simulink model "rlDronePidTuning"  (R2024b)
settings: Solver=VariableStepAuto  StartTime=0.0  StopTime=60  RelTol=1e-3
libraries: simulink x5, rllib x1
settings Model: Creator=Feder  LastModifiedBy=Alessandro
settings DataIOCC: ReturnWorkspaceOutputs=off
settings DebuggingCC: AlgebraicLoopMsg=none

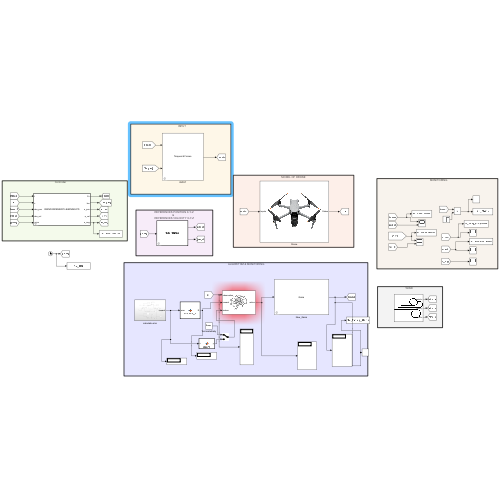
[thumbnail: Simulink's stored preview of the top-level diagram]
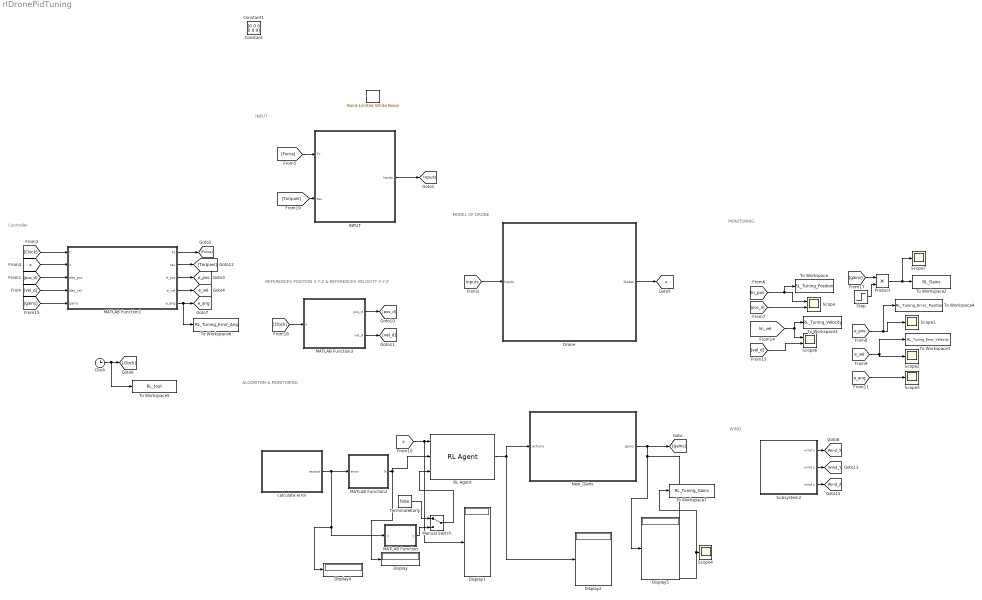
== system rlDronePidTuning ==
  note: MONITORING
  note: ALGORITHM & MONITORING
  note: Controller
  note: REFERENCES POSITION X-Y-Z
      |                                                 &
      |                         REFERENCES VELOCITY X-Y-Z
  note: INPUT
  note: MODEL OF DRONE
  note: WIND
  Clock : Clock
  Display{,1..2,4..5} (5 alike) : Display
  Drone : Subsystem
      mask Display: image('DJI Air 3S.png');
  INPUT : Subsystem
      mask Display: disp('Torques & Forces');
  MATLAB Function : MATLAB Function  TreatAsAtomicUnit=on
  MATLAB Function1 : MATLAB Function  TreatAsAtomicUnit=on
  MATLAB Function2 : MATLAB Function  TreatAsAtomicUnit=on
  MATLAB Function3 : MATLAB Function  TreatAsAtomicUnit=on
  Manual Switch : ManualSwitch
  New_Gains : Subsystem
      mask Display: disp('Gains');
  Product : Product
  RL Agent : rllib/RL Agent  Agent=myAgent  ExternalActionAsInput=off  ProvideLastAction=off  ProvideCumRwd=off  TreatAsDirectFeedthrough=on  UseStrictObservationDataTypes=off
  Scope : Scope  NumInputPorts=2
  Scope{1..4,7} (5 alike) : Scope
  Scope6 : Scope  NumInputPorts=2
  Step : Step  Time=0  SampleTime=0
  Subsystem2 : Subsystem
      mask Display: image('wind-14.png');
  TerminateEarly : Constant  Value=false
  To Workspace : ToWorkspace  VariableName=RL_Tuning_Position  SampleTime=-1
  To Workspace1 : ToWorkspace  VariableName=RL_Tuning_Velocity  SampleTime=-1
  To Workspace2 : ToWorkspace  VariableName=RL_Gains  SampleTime=-1
  To Workspace3 : ToWorkspace  VariableName=RL_Tuning_Error_Velocity  SampleTime=-1
  To Workspace4 : ToWorkspace  VariableName=RL_Tuning_Error_Position  SampleTime=-1
  To Workspace5 : ToWorkspace  VariableName=RL_tout  SampleTime=-1
  To Workspace6 : ToWorkspace  VariableName=RL_Tuning_Error_Ang  SampleTime=-1
  To Workspace7 : ToWorkspace  VariableName=RL_Tuning_Gains  SaveFormat=Timeseries  SampleTime=-1
  calculate error : Subsystem
  " " : simulink/Sources/Band-Limited White Noise  IOType=siggen  Cov=[0.1]  Ts=0.1  seed=[23341]
      settings: LibrarySourceBlock=|
      | simgens/Band-Limited
      | White Noise
  Constant : Constant  IOType=siggen
  Constant1 : Constant  IOType=siggen  Value=[0 0 0 0 0 0]
  tag scope: Inputs=global, Wind_X=global, Wind_Y=global, Wind_Z=global, e_ang=global, e_pos=global, e_vel=global, x=global
  wires:
  MATLAB Function1/3(e_pos) -> [e_pos]
  MATLAB Function1/4(e_vel) -> [e_vel]
  [x] -> MATLAB Function1/2(x)
  [vel_d] -> MATLAB Function1/4(des_vel)
  [pos_d] -> MATLAB Function1/3(des_pos)
  Clock/1 -> To Workspace5/1, [Clock]
  [Clock] -> MATLAB Function1/1(t)
  [lin_pos] -> Scope/1, To Workspace/1
  [pos_d] -> Scope/2
  MATLAB Function2/1(R) -> Display/1, RL Agent/2
  [x] -> Display1/1, RL Agent/1
  [vel_d] -> Scope6/2
  [lin_vel] -> To Workspace1/1, Scope6/1
  Step/1 -> Product/2
  Product/1 -> To Workspace2/1, Scope7/1
  [gains] -> MATLAB Function1/5(gains)
  [gains] -> Product/1
  [e_pos] -> To Workspace4/1, Scope1/1
  [e_vel] -> To Workspace3/1, Scope2/1
  [e_ang] -> Scope3/1
  [Clock] -> MATLAB Function3/1(t)
  MATLAB Function3/2(vel_d) -> [vel_d]
  MATLAB Function3/1(pos_d) -> [pos_d]
  [Force] -> INPUT/1(Fz)
  [Torques] -> INPUT/2(tau)
  INPUT/1(Inputs) -> [Inputs]
  MATLAB Function1/1(Fz) -> [Force]
  MATLAB Function1/2(tau) -> [Torques]
  MATLAB Function1/5(e_ang) -> To Workspace6/1, [e_ang]
  Drone/1(States) -> [x]
  [Inputs] -> Drone/1(Inputs)
  Subsystem2/2(wind y) -> [Wind_Y]
  Subsystem2/1(wind x) -> [Wind_X]
  Subsystem2/3(wind z) -> [Wind_Z]
  New_Gains/1(gains) -> [gains], To Workspace7/1, Scope4/1, Display5/1
  RL Agent/1 -> Display2/1, New_Gains/1(actions)
  calculate error/1(reward) -> MATLAB Function/1(u), Display4/1, MATLAB Function2/1(error)
  TerminateEarly/1 -> Manual Switch/1
  MATLAB Function/1(y) -> Manual Switch/2
  Manual Switch/1 -> RL Agent/3

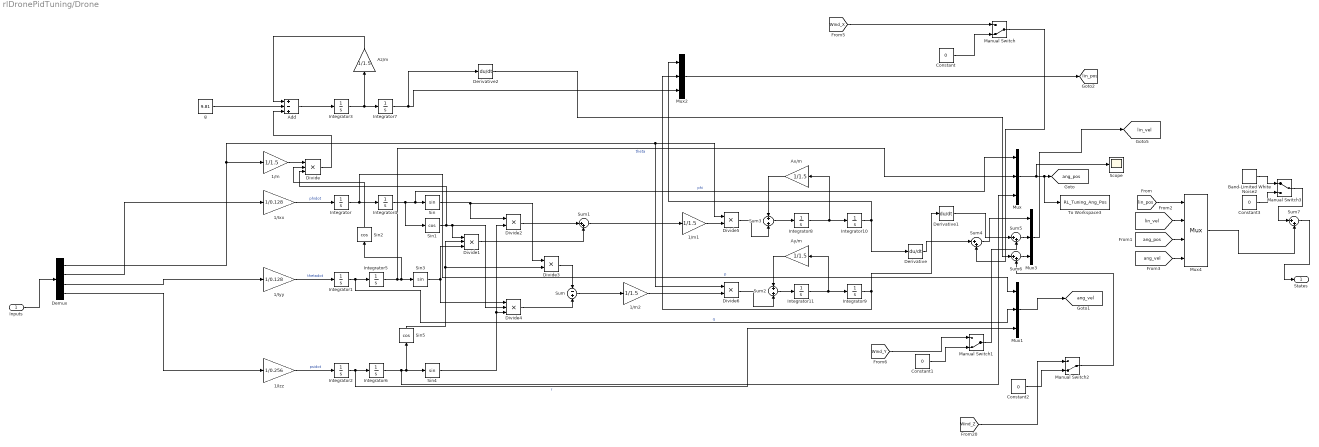
== system rlDronePidTuning/Drone ==
  Inputs : Inport
  1/Ixx : Gain  Gain=1/0.128
  1/Iyy : Gain  Gain=1/0.128
  1/Izz : Gain  Gain=1/0.256
  1/m : Gain  Gain=1/1.5
  1/m1 : Gain  Gain=1/1.5
  1/m2 : Gain  Gain=1/1.5
  Add : Sum  Inputs=+-+
  Ax/m : Gain  Gain=1/1.5
  Ay/m : Gain  Gain=1/1.5
  Az/m : Gain  Gain=1/1.5
  Band-Limited White Noise2 : simulink/Sources/Band-Limited White Noise  Cov=[0.00001]  Ts=0.01  seed=[23341]
  Constant{,1..3} (4 alike) : Constant  Value=0
  Demux : Demux
  Derivative : Derivative
  Derivative1 : Derivative
  Derivative2 : Derivative
  Divide : Product  Inputs=***
  Divide1 : Product  Inputs=***
  Divide{2..3,5..6} (4 alike) : Product  Inputs=**
  Divide4 : Product  Inputs=***
  Integrator{,1..11} (12 alike) : Integrator
  Manual Switch : ManualSwitch  CurrentSetting=0
  Manual Switch1 : ManualSwitch  CurrentSetting=0
  Manual Switch2 : ManualSwitch  CurrentSetting=0
  Manual Switch3 : ManualSwitch
  Mux{,1..3} (4 alike) : Mux  Inputs=3
  Mux4 : Mux
  Scope : Scope
  Sin : Trigonometry
  Sin1 : Trigonometry  Operator=cos
  Sin2 : Trigonometry  Operator=cos
  Sin3 : Trigonometry
  Sin4 : Trigonometry
  Sin5 : Trigonometry  Operator=cos
  Sum : Sum  Inputs=-+
  Sum{1,4..7} (5 alike) : Sum  Inputs=|++
  Sum2 : Sum
  Sum3 : Sum
  To Workspace3 : ToWorkspace  VariableName=RL_Tuning_Ang_Pos  SampleTime=-1
  g : Constant  Value=9.81
  States : Outport
  tag scope: ang_pos=global, ang_vel=global, lin_pos=global, lin_vel=global
  wires:
  Ay/m/1 -> Sum2/1
  Sum3/1 -> Integrator8/1
  Divide2/1 -> Sum1/1
  Integrator5/1 -> Mux/2, Sin2/1, Sin3/1  "theta"
  Ax/m/1 -> Sum3/1
  Integrator2/1 -> Mux1/3, Integrator6/1  "r"
  Demux/1 -> Divide6/1, Divide5/1, 1/m/1
  Integrator11/1 -> Ay/m/1, Integrator9/1
  Divide1/1 -> Sum1/2
  1/Izz/1 -> Integrator2/1  "psidot"
  Divide6/1 -> Sum2/2
  Divide5/1 -> Sum3/2
  Sum/1 -> 1/m2/1
  Integrator6/1 -> Mux/3, Sin5/1, Sin4/1
  Az/m/1 -> Add/1
  Integrator3/1 -> Az/m/1, Integrator7/1
  Divide/1 -> Add/3
  Integrator/1 -> Mux1/1, Integrator4/1  "p"
  Sin4/1 -> Divide2/2, Divide4/3
  Integrator10/1 -> Mux2/1, Derivative/1
  Divide4/1 -> Sum/2
  1/Ixx/1 -> Integrator/1  "phidot"
  Add/1 -> Integrator3/1
  Integrator9/1 -> Derivative1/1, Mux2/2
  Divide3/1 -> Sum/1
  1/Iyy/1 -> Integrator1/1  "thetadot"
  Sin/1 -> Divide2/1, Divide3/1
  1/m2/1 -> Divide6/2
  Integrator1/1 -> Mux1/2, Integrator5/1  "q"
  Sin2/1 -> Divide/2
  Sin5/1 -> Divide1/2, Divide3/2
  Sum2/1 -> Integrator11/1
  Integrator4/1 -> Mux/1, Sin/1, Sin1/1  "phi"
  Sin1/1 -> Divide/3, Divide1/1, Divide4/2
  g/1 -> Add/2
  1/m/1 -> Divide/1
  Sin3/1 -> Divide4/1, Divide1/3
  Sum1/1 -> 1/m1/1
  1/m1/1 -> Divide5/2
  Integrator8/1 -> Ax/m/1, Integrator10/1
  Mux/1 -> Scope/1, To Workspace3/1, [ang_pos]
  Mux1/1 -> [ang_vel]
  Integrator7/1 -> Derivative2/1, Mux2/3
  [lin_pos] -> Mux4/1
  [ang_pos] -> Mux4/3
  [lin_vel] -> Mux4/2
  [ang_vel] -> Mux4/4
  Demux/2 -> 1/Ixx/1
  Demux/3 -> 1/Iyy/1
  Demux/4 -> 1/Izz/1
  Inputs/1 -> Demux/1
  Mux2/1 -> [lin_pos]
  Mux3/1 -> [lin_vel]
  [Wind_X] -> Manual Switch/1
  Constant/1 -> Manual Switch/2
  Manual Switch/1 -> Sum4/2
  Derivative/1 -> Sum4/1
  Sum4/1 -> Mux3/1
  Derivative1/1 -> Sum5/1
  Sum5/1 -> Mux3/2
  Constant1/1 -> Manual Switch1/2
  [Wind_Y] -> Manual Switch1/1
  Manual Switch1/1 -> Sum5/2
  Sum6/1 -> Mux3/3
  Derivative2/1 -> Sum6/1
  [Wind_Z] -> Manual Switch2/1
  Constant2/1 -> Manual Switch2/2
  Manual Switch2/1 -> Sum6/2
  Sum7/1 -> States/1
  Mux4/1 -> Sum7/2
  Band-Limited White Noise2/1 -> Manual Switch3/1
  Constant3/1 -> Manual Switch3/2
  Manual Switch3/1 -> Sum7/1

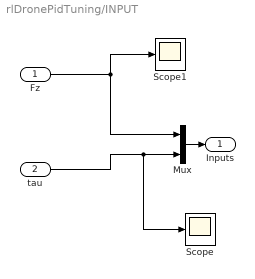
== system rlDronePidTuning/INPUT ==
  Fz : Inport
  tau : Inport  Port=2
  Mux : Mux  Inputs=2
  Scope : Scope
  Scope1 : Scope
  Inputs : Outport
  wires:
  Fz/1 -> Mux/1, Scope1/1
  Mux/1 -> Inputs/1
  tau/1 -> Scope/1, Mux/2

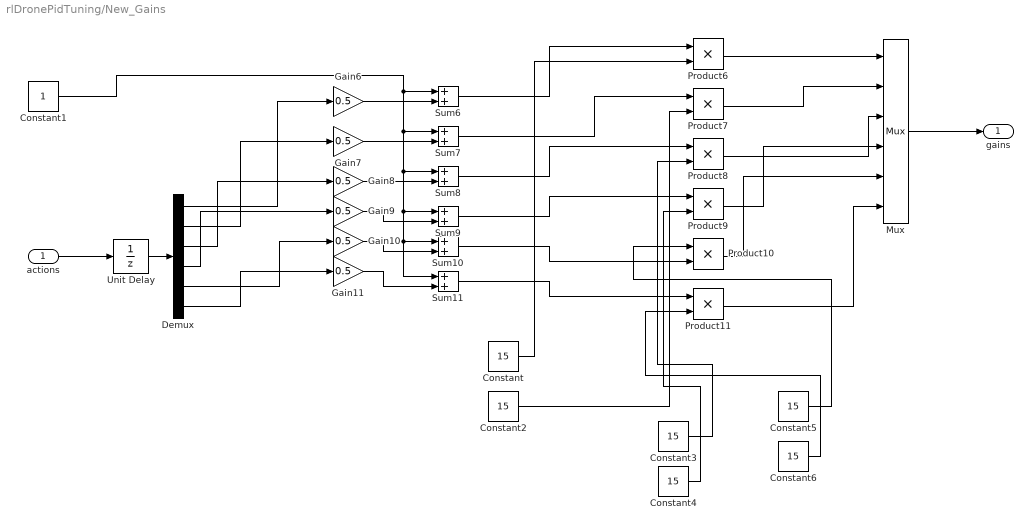
== system rlDronePidTuning/New_Gains ==
  actions : Inport
  Constant{,2..6} (6 alike) : Constant  Value=15
  Constant1 : Constant
  Demux : Demux  Outputs=6
  Gain{6..11} (6 alike) : Gain  Gain=0.5
  Mux : Mux  Inputs=6
  Product{6..11} (6 alike) : Product
  Sum{6..11} (6 alike) : Sum
  Unit Delay : UnitDelay  SampleTime=-1  HasFrameUpgradeWarning=on
  gains : Outport
  wires:
  Gain10/1 -> Sum10/2
  Sum10/1 -> Product10/2
  Gain8/1 -> Sum8/2
  Sum11/1 -> Product11/1
  Sum6/1 -> Product6/1
  Sum8/1 -> Product8/1
  Gain6/1 -> Sum6/2
  Sum7/1 -> Product7/1
  Constant1/1 -> Sum11/1, Sum10/1, Sum9/1, Sum8/1, Sum7/1, Sum6/1
  Gain11/1 -> Sum11/2
  Gain9/1 -> Sum9/2
  Sum9/1 -> Product9/1
  Gain7/1 -> Sum7/2
  Demux/3 -> Gain8/1
  Demux/5 -> Gain10/1
  Demux/2 -> Gain7/1
  Unit Delay/1 -> Demux/1
  Demux/4 -> Gain9/1
  Demux/6 -> Gain11/1
  Demux/1 -> Gain6/1
  actions/1 -> Unit Delay/1
  Constant/1 -> Product6/2
  Constant2/1 -> Product7/2
  Constant3/1 -> Product8/2
  Constant4/1 -> Product9/2
  Constant5/1 -> Product10/1
  Constant6/1 -> Product11/2
  Product6/1 -> Mux/1
  Product9/1 -> Mux/4
  Product11/1 -> Mux/6
  Mux/1 -> gains/1
  Product8/1 -> Mux/3
  Product10/1 -> Mux/5
  Product7/1 -> Mux/2

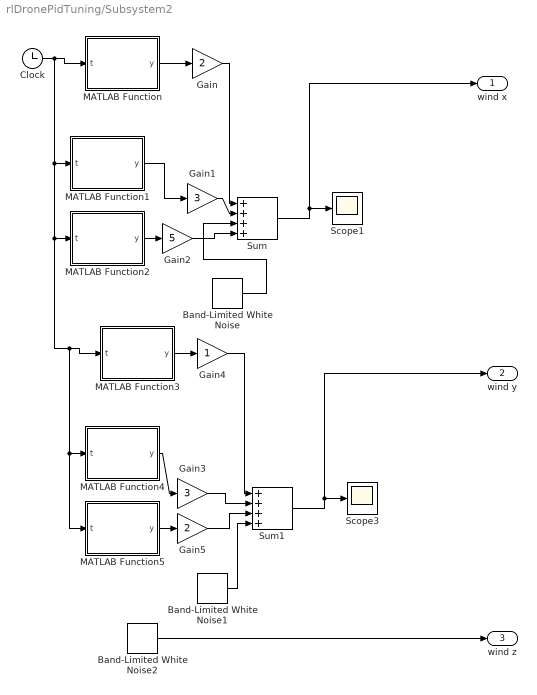
== system rlDronePidTuning/Subsystem2 ==
  Band-Limited White Noise : simulink/Sources/Band-Limited White Noise  Cov=[0.00001]  Ts=0.01  seed=[23341]
  Band-Limited White Noise1 : simulink/Sources/Band-Limited White Noise  Cov=[0.000001]  Ts=0.01  seed=[23341]
  Band-Limited White Noise2 : simulink/Sources/Band-Limited White Noise  Cov=[0.00001]  Ts=0.01  seed=[23341]
  Clock : Clock
  Gain : Gain  Gain=2
  Gain1 : Gain  Gain=3
  Gain2 : Gain  Gain=5
  Gain3 : Gain  Gain=3
  Gain4 : Gain
  Gain5 : Gain  Gain=2
  MATLAB Function : MATLAB Function  TreatAsAtomicUnit=on
  MATLAB Function1 : MATLAB Function  TreatAsAtomicUnit=on
  MATLAB Function2 : MATLAB Function  TreatAsAtomicUnit=on
  MATLAB Function3 : MATLAB Function  TreatAsAtomicUnit=on
  MATLAB Function4 : MATLAB Function  TreatAsAtomicUnit=on
  MATLAB Function5 : MATLAB Function  TreatAsAtomicUnit=on
  Scope1 : Scope
  Scope3 : Scope
  Sum : Sum  Inputs=++++
  Sum1 : Sum  Inputs=++++
  wind x : Outport
  wind y : Outport  Port=2
  wind z : Outport  Port=3
  wires:
  MATLAB Function/1(y) -> Gain/1
  Gain/1 -> Sum/1
  Sum/1 -> wind x/1, Scope1/1
  Gain1/1 -> Sum/2
  MATLAB Function1/1(y) -> Gain1/1
  MATLAB Function2/1(y) -> Gain2/1
  Gain2/1 -> Sum/4
  Clock/1 -> MATLAB Function5/1(t), MATLAB Function4/1(t), MATLAB Function3/1(t), MATLAB Function2/1(t), MATLAB Function1/1(t), MATLAB Function/1(t)
  MATLAB Function3/1(y) -> Gain4/1
  Sum1/1 -> wind y/1, Scope3/1
  MATLAB Function5/1(y) -> Gain5/1
  Gain4/1 -> Sum1/1
  MATLAB Function4/1(y) -> Gain3/1
  Gain3/1 -> Sum1/2
  Gain5/1 -> Sum1/3
  Band-Limited White Noise/1 -> Sum/3
  Band-Limited White Noise1/1 -> Sum1/4
  Band-Limited White Noise2/1 -> wind z/1

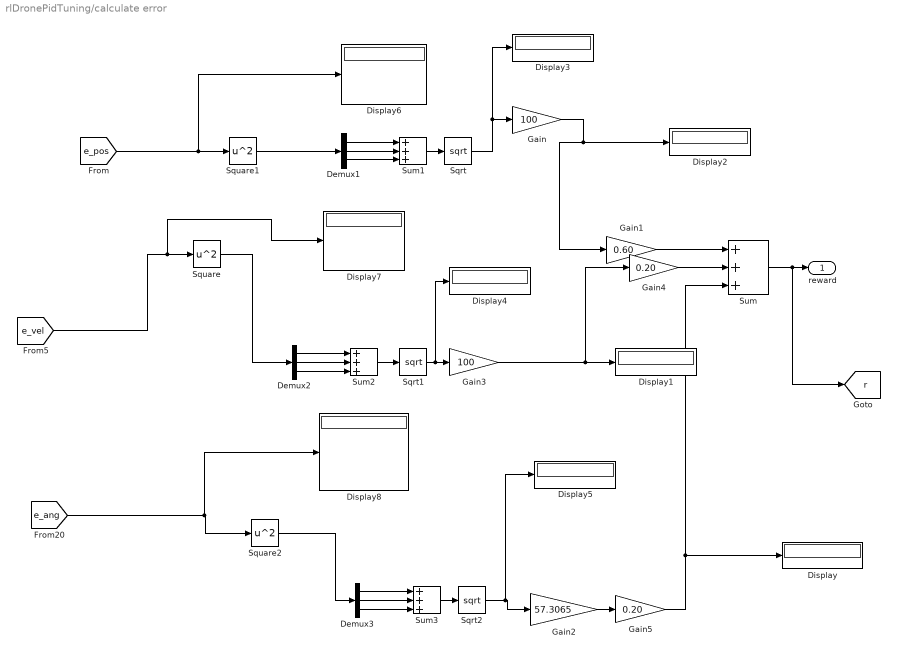
== system rlDronePidTuning/calculate error ==
  Demux1 : Demux  Outputs=3
  Demux2 : Demux  Outputs=3
  Demux3 : Demux  Outputs=3
  Display{,1..8} (9 alike) : Display
  Gain : Gain  Gain=100
  Gain1 : Gain  Gain=0.60
  Gain2 : Gain  Gain=57.3065
  Gain3 : Gain  Gain=100
  Gain4 : Gain  Gain=0.20
  Gain5 : Gain  Gain=0.20
  Sqrt : Sqrt
  Sqrt1 : Sqrt
  Sqrt2 : Sqrt
  Square : Math  Operator=square
  Square1 : Math  Operator=square
  Square2 : Math  Operator=square
  Sum{,1..3} (4 alike) : Sum  Inputs=+++
  reward : Outport  VectorParamsAs1DForOutWhenUnconnected=off
  tag scope: r=global
  wires:
  [e_pos] -> Display6/1, Square1/1
  [e_vel] -> Display7/1, Square/1
  Square/1 -> Demux2/1
  Demux2/1 -> Sum2/1
  Demux2/2 -> Sum2/2
  Demux2/3 -> Sum2/3
  Sum2/1 -> Sqrt1/1
  Demux1/3 -> Sum1/3
  Demux1/1 -> Sum1/1
  Square1/1 -> Demux1/1
  Demux1/2 -> Sum1/2
  Gain/1 -> Gain1/1, Display2/1
  Sum/1 -> [r], reward/1
  Demux3/1 -> Sum3/1
  Square2/1 -> Demux3/1
  Demux3/2 -> Sum3/2
  [e_ang] -> Display8/1, Square2/1
  Demux3/3 -> Sum3/3
  Gain2/1 -> Gain5/1
  Sum1/1 -> Sqrt/1
  Sqrt/1 -> Display3/1, Gain/1
  Sqrt1/1 -> Display4/1, Gain3/1
  Gain3/1 -> Gain4/1, Display1/1
  Sum3/1 -> Sqrt2/1
  Sqrt2/1 -> Display5/1, Gain2/1
  Gain1/1 -> Sum/1
  Gain4/1 -> Sum/2
  Gain5/1 -> Sum/3, Display/1

== matlab function rlDronePidTuning/Subsystem2/MATLAB Function5 ==
  data: t input; y output
function y = bell(t)
%#codegen
y = exp(-((t - 30).^2) / (7*2^2));

== matlab function rlDronePidTuning/MATLAB Function ==
  data: u input; y output
function y = isDone(u)

if u > 200
    y =1;
else 
    y = 0;
end

== matlab function rlDronePidTuning/MATLAB Function1 ==
  data: t input; Fz output; x input; des_pos input; des_vel input; tau output; e_pos output; e_vel output; gains input; e_ang output
function [Fz, tau,e_pos,e_vel,e_ang]  = PID_controller(t, x, des_pos, des_vel,gains)
   



    g = 9.81;
    Kp = diag([gains(1) ,  gains(3), gains(5)]); 
    Kd = diag([gains(2), gains(4),   gains(6)]);
    Kp_ang = diag([150, 150, 100]);
    Kd_ang = diag([50, 50, 30]);
    m = 1.15;

    pos = x(1:3);
    vel = x(4:6);
    phi = x(7);
    theta = x(8);
    psi = x(9);
    omega = x(10:12);
    
    % === Controllo posizione ===
    e_pos = des_pos - pos;
    e_vel = des_vel - vel;
    acc_des = Kp * e_pos + Kd * e_vel;
    
    % Forza lungo z
    Fz = m * (acc_des(3) + g);
    
    % === Controllo orientamento ===
    phi_des   = (1/g)*(acc_des(1)*sin(psi) - acc_des(2)*cos(psi));
    theta_des = (1/g)*(acc_des(1)*cos(psi) + acc_des(2)*sin(psi));
    psi_des   = 0;  % fissa per semplicità
    
    ang_des = [phi_des; theta_des; psi_des];
    ang     = [phi; theta; psi];
    
    e_ang   = ang_des - ang;
    e_omega = -omega; % si può modificare se hai riferimento su omega
    
    tau = Kp_ang * e_ang + Kd_ang * e_omega;
end

== matlab function rlDronePidTuning/Subsystem2/MATLAB Function ==
  data: t input; y output
function y = bell(t)
%#codegen
y = exp(-((t - 10).^2) / (6*2^2));

== matlab function rlDronePidTuning/MATLAB Function2 ==
  data: error input; R output
function R = calculate_R(error)
    if error >= 11.5
        R = -25;
    elseif error >= 10.5 && error < 11.5
        R = -15;
    elseif error >= 9.5 && error < 10.5
        R = -10;
    elseif error >= 8.5 && error < 9.5
        R = -5;
    elseif error >= 7.5 && error < 8.5
        R = -1;
    elseif error >= 6.5 && error < 7.5
        R = 10
    else
        R = 15;
    end
end

== matlab function rlDronePidTuning/MATLAB Function3 ==
  data: t input; pos_d output; vel_d output
function [pos_d, vel_d] = reference_trajectory(t)
   % Aggiungi all'inizio della funzione quadrotor_ode:
pos_d = [t; sin(0.5*t); 2 + 0.5*cos(0.5*t)];
vel_d = [1; 0.5*cos(0.5*t); -0.25*sin(0.5*t)];

end

== matlab function rlDronePidTuning/Subsystem2/MATLAB Function1 ==
  data: t input; y output
function y = bell(t)
%#codegen
y = exp(-((t - 17).^2) / (0.5*2^2));

== matlab function rlDronePidTuning/Subsystem2/MATLAB Function2 ==
  data: t input; y output
function y = bell(t)
%#codegen
y = exp(-((t - 35).^2) / (7*2^2));

== matlab function rlDronePidTuning/Subsystem2/MATLAB Function3 ==
  data: t input; y output
function y = bell(t)
%#codegen
y = exp(-((t - 32).^2) / (7*2^2));

== matlab function rlDronePidTuning/Subsystem2/MATLAB Function4 ==
  data: t input; y output
function y = bell(t)
%#codegen
y = exp(-((t - 37).^2) / (3*2^2));
